simulink model "data_record"  (R2018b)
settings: Solver=ode4  StartTime=0.0  StopTime=inf  FixedStep=1/120  RelTol=1e-3
libraries: instrumentlib x2, vrlib x1, robotcorelib x1, simulink x1
settings Model: Creator=pprz  LastModifiedBy=pprz
settings DebuggingCC: LibraryContextMissingDiagnostic=none
settings SFSimCC: SimUseLocalCustomCode=off
settings RTWCC: RTWUseLocalCustomCode=off

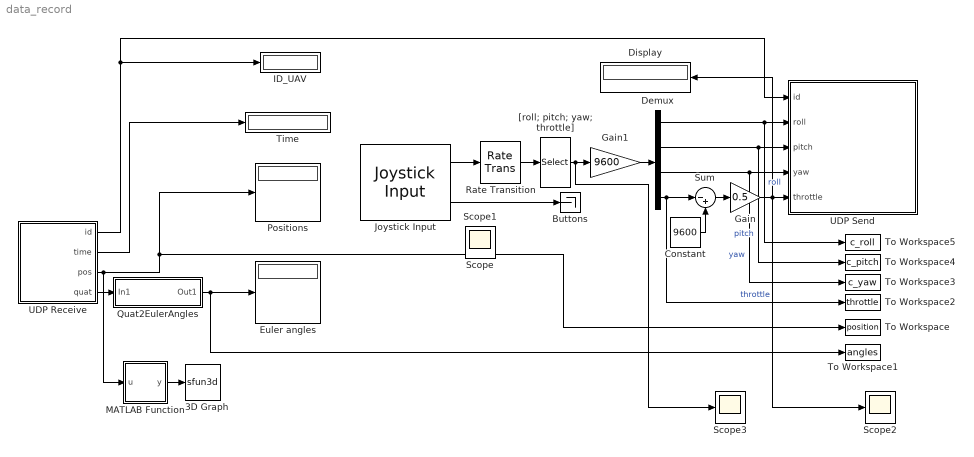
== system data_record ==
  3D Graph : S-Function  LoadFcn=if exist('sfun3d','file'), sfun3d([],[],[],'LoadBlock'); end  FunctionName=sfun3d  Parameters=ax,T,np,cp,gd,ls,mk,mx,hd,tb  SFunctionDeploymentMode=off  EnableBusSupport=off  mask(3D Graph){np=1, ax=[-3 3 -3 3 0 3], mx=1e4, T=0.1, cp=[3 2 1], gd=on, hd=on, tb=on, ls=-, mk=none}
      mask prompts: np "Number of moving points (lines)"; ax "Range: [xmin xmax  ymin ymax zmin zmax]"; mx "Max number of points in each line"; T "Sampling Time"; cp "Camera position (use [0 0 1] for 2D XY view)"; gd "Grid (on|off)"; hd "HeadMarkers (on|off)"; tb "Toolbar (on|off)"; ls "LineStyle"; mk "LineMarker"
      mask help:
      | This block plots the position of several points in the XYZ space. The input contains the coordinates of all the points (x1,y1,z1,x2,y2,z2,...).
      | The number of moving points (lines), the XYZ ranges, sampling time, camera position, and grid (among other things) can be set as mask parameters.
      settings: CopyFcn=if exist('sfun3d','file'), sfun3d([],[],[],'CopyBlock'); end  DeleteFcn=if exist('sfun3d','file'), sfun3d([],[],[],'DeleteBlock'); end  NameChangeFcn=if exist('sfun3d','file'), sfun3d([],[],[],'NameChange'); end
      mask Help:
      | This block plots the position of several points in the XYZ space. The input contains the coordinates of all the points (x1,y1,z1,x2,y2,z2,...).
      | The number of moving points (lines), the XYZ ranges, sampling time, camera position, and grid (among other things) can be set as mask parameters.
      mask TypeOptions ls: - | -- | : | -. | none
      mask TypeOptions mk: none | . | + | o | * | x | square | diamond | v | ^ | > | < | pentagram | hexagram
      mask Display: plot([.05 .95 .95 .05 .05],[.45 .45 .95 .95 .45], 0.5+cos(0:0.1:2*pi)*0.3,0.7+sin(0:0.1:2*pi)*0.2)
  Buttons : Terminator
  Constant : Constant  Value=9600
  Demux : Demux
  Display : Display
  Euler angles : Display
  Gain : Gain  Gain=0.5
  Gain1 : Gain  Gain=9600  OutDataTypeStr=Inherit: Same as input
  ID_UAV : Display
  Joystick Input : vrlib/Joystick Input  joyid=1  adjustports=on  forcefeed=off
      settings: SourceProductBaseCode=VR
  MATLAB Function : MATLAB Function  TreatAsAtomicUnit=on
  Positions : Display
  Quat2EulerAngles : Subsystem
  Rate Transition : RateTransition  OutPortSampleTime=1/120
  Scope{,1..3} (4 alike) : Scope
  Sum : Sum  Inputs=|-+
  Time : Display
  To Workspace : ToWorkspace  VariableName=position  SaveFormat=Structure With Time  SampleTime=-1
  To Workspace1 : ToWorkspace  VariableName=angles  SaveFormat=Structure With Time  SampleTime=-1
  To Workspace2 : ToWorkspace  VariableName=throttle  SaveFormat=Structure With Time  SampleTime=-1
  To Workspace3 : ToWorkspace  VariableName=c_yaw  SaveFormat=Structure With Time  SampleTime=-1
  To Workspace4 : ToWorkspace  VariableName=c_pitch  SaveFormat=Structure With Time  SampleTime=-1
  To Workspace5 : ToWorkspace  VariableName=c_roll  SaveFormat=Structure With Time  SampleTime=-1
  UDP Receive : Subsystem  mask(Natnet/PPRZ UDP receiver){Host=huppe, Port=9090, LocalPort=5005, out_freq=10}
      mask prompts: Host "Remote Host"; Port "Remote Port"; LocalPort "Local port"; out_freq "Output frequency"
      mask help: Receive position and orientation from PPRZ Natnet bridge
      mask TypeOptions Host: UDP Receive/Host
      mask TypeOptions Port: UDP Receive/Port
      mask TypeOptions LocalPort: UDP Receive/LocalPort
      mask Display: image('penguin_logo.gif');
  UDP Send : Subsystem  mask(PPRZ UDP sender){Host=192.168.1.236, Port=9090, out_freq=10}
      mask prompts: Host "Remote Host"; Port "Remote Port"; out_freq "Output freq"
      mask help: Send ID and commands to PPRZ Ivy bridge
      mask TypeOptions Host: UDP Send/Host
      mask TypeOptions Port: UDP Send/Port
      mask Display: image('penguin_logo.gif');
  "[roll; pitch; yaw; throttle]" : Selector  InputPortWidth=6  IndexOptions=Index vector (dialog)  Indices=[1 2 3 4]  OutputSizes=1
  wires:
  UDP Receive/2(time) -> Time/1
  UDP Receive/1(id) -> UDP Send/1(id), ID_UAV/1
  Joystick Input/2 -> Buttons/1
  Demux/1 -> To Workspace5/1, UDP Send/2(roll)  "roll"
  "[roll; pitch; yaw; throttle]"/1 -> Scope3/1, Gain1/1
  Gain1/1 -> Demux/1
  Demux/2 -> UDP Send/3(pitch), To Workspace4/1  "pitch"
  Demux/3 -> To Workspace3/1, UDP Send/4(yaw)  "yaw"
  Constant/1 -> Sum/2
  Demux/4 -> Sum/1, To Workspace2/1  "throttle"
  Sum/1 -> Gain/1
  Gain/1 -> Display/1, Scope2/1, UDP Send/5(throttle)
  UDP Receive/3(pos) -> MATLAB Function/1(u), Positions/1, To Workspace/1
  MATLAB Function/1(y) -> 3D Graph/1
  Quat2EulerAngles/1(Out1) -> Euler angles/1, To Workspace1/1
  UDP Receive/4(quat) -> Quat2EulerAngles/1(In1)
  Joystick Input/1 -> Rate Transition/1
  Rate Transition/1 -> "[roll; pitch; yaw; throttle]"/1

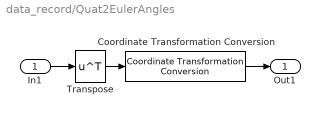
== system data_record/Quat2EulerAngles ==
  In1 : Inport
  Coordinate Transformation Conversion : robotcorelib/Coordinate Transformation Conversion  InputRepresentation=Quaternion  InputEulerSequence=ZYX  ShowTrVecInputPort=on  OutputRepresentation=Euler Angles  OutputEulerSequence=ZYX  ShowTrVecOutputPort=on  SimulateUsing=Interpreted execution
      settings: SourceProductBaseCode=RO
  Transpose : Math  Operator=transpose  SaturateOnIntegerOverflow=on
  Out1 : Outport
  wires:
  Transpose/1 -> Coordinate Transformation Conversion/1
  In1/1 -> Transpose/1
  Coordinate Transformation Conversion/1 -> Out1/1

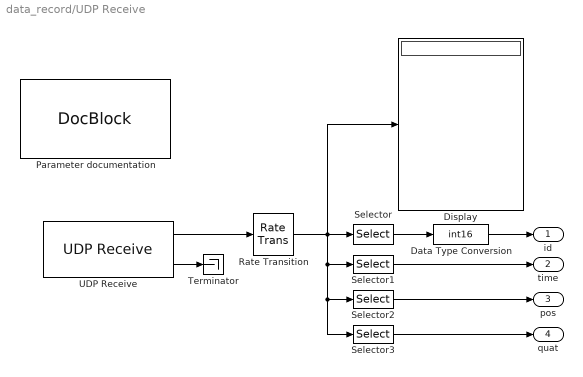
== system data_record/UDP Receive ==
  Data Type Conversion : DataTypeConversion  OutDataTypeStr=int16
  Display : Display
  Parameter documentation : simulink/Model-Wide Utilities/DocBlock  Description=Note on parameters  DocumentType=Text
      content=|
      | The remote port parameter is unused.
      | You need to set LocalPort to the port you want to receive data to.
      | You need to set the Remote Address to the address of the machine that sends
      | the data or to 0.0.0.0 to remove filtering on data source.
  Rate Transition : RateTransition  OutPortSampleTime=1/out_freq
  Selector : Selector  InputPortWidth=9  IndexOptions=Index vector (dialog)  Indices=[1]  OutputSizes=1
  Selector1 : Selector  InputPortWidth=9  IndexOptions=Index vector (dialog)  Indices=[2]  OutputSizes=1
  Selector2 : Selector  InputPortWidth=9  IndexOptions=Index vector (dialog)  Indices=[3 4 5]  OutputSizes=1
  Selector3 : Selector  InputPortWidth=9  IndexOptions=Index vector (dialog)  Indices=[6 7 8 9]  OutputSizes=1
  Terminator : Terminator
  UDP Receive : instrumentlib/UDP Receive  Host=huppe  Port=Port  LocalPort=LocalPort  EnablePortSharing=off  GetLatestData=off  DataSize="[1  9]"  DataType=single  ASCIIFormatting=%f  Terminator=LF  ByteOrder=LittleEndian  EnableBlockingMode=off  Timeout=10  SampleTime=-1  LocalAddress=0.0.0.0
      settings: SourceProductName=Instrument Control Toolbox
  id : Outport  OutDataTypeStr=int16
  time : Outport  Port=2
  pos : Outport  Port=3
  quat : Outport  Port=4
  wires:
  UDP Receive/1 -> Rate Transition/1
  Selector/1 -> Data Type Conversion/1
  Selector1/1 -> time/1
  Selector2/1 -> pos/1
  Selector3/1 -> quat/1
  UDP Receive/2 -> Terminator/1
  Data Type Conversion/1 -> id/1
  Rate Transition/1 -> Selector3/1, Selector2/1, Selector1/1, Display/1, Selector/1

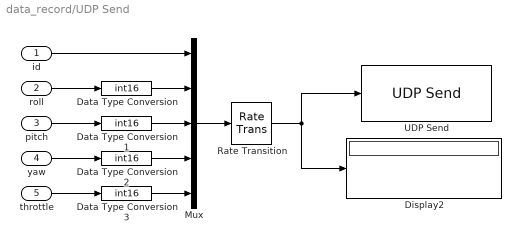
== system data_record/UDP Send ==
  id : Inport  OutDataTypeStr=int16
  roll : Inport  Port=2
  pitch : Inport  Port=3
  yaw : Inport  Port=4
  throttle : Inport  Port=5
  Data Type Conversion{,1..3} (4 alike) : DataTypeConversion  OutDataTypeStr=int16
  Display2 : Display
  Mux : Mux  Inputs=5
  Rate Transition : RateTransition  OutPortSampleTime=1/out_freq
  UDP Send : instrumentlib/UDP Send  Host=192.168.1.236  Port=Port  LocalPort=-1  EnablePortSharing=off  ByteOrder=LittleEndian  OutputDatagramPacketSize=10  EnableBlockingMode=on  LocalAddress=0.0.0.0
      settings: SourceProductName=Instrument Control Toolbox
  wires:
  Mux/1 -> Rate Transition/1
  throttle/1 -> Data Type Conversion3/1
  yaw/1 -> Data Type Conversion2/1
  pitch/1 -> Data Type Conversion1/1
  id/1 -> Mux/1
  Data Type Conversion/1 -> Mux/2
  Data Type Conversion1/1 -> Mux/3
  Data Type Conversion2/1 -> Mux/4
  Data Type Conversion3/1 -> Mux/5
  roll/1 -> Data Type Conversion/1
  Rate Transition/1 -> Display2/1, UDP Send/1

== matlab function data_record/MATLAB Function ==
  data: u input; y output
function y = fcn(u)

y = double(u);
